simulink model "bh_smd_MAIN_HELLO"  (R2018a)
settings: Solver=ode45  StartTime=0.0  StopTime=10.0  RelTol=1e-7
settings Model: Creator=bhorton  LastModifiedBy=bhorton
settings CodeAppCC: StateflowObjectComments=on

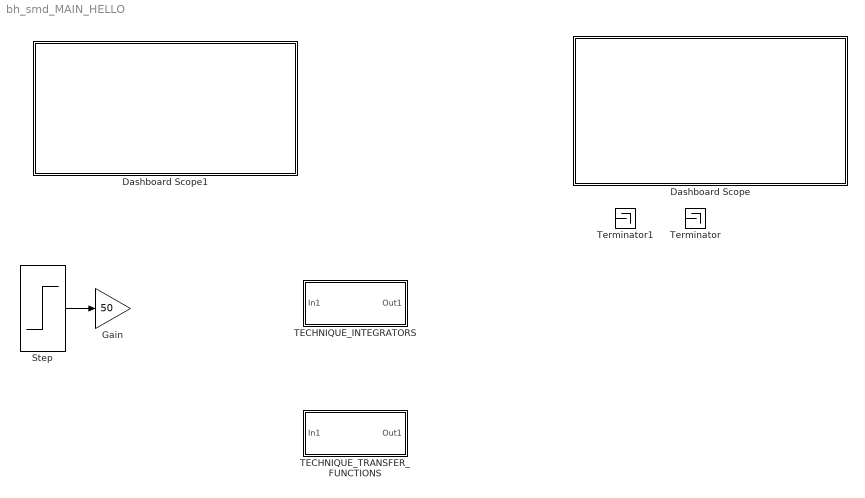
== system bh_smd_MAIN_HELLO ==
  Dashboard Scope : Subsystem  DialogController=hmiCreateDDGDialog  IsWebBlock=on  mask(MWDashboardBlock){webBlockId=47d7a76a-e090-4f37-bb13-c45fee118520, webBlockType=sdiscope, ShowInitialText=on, HMISrcModelName=bh_smd_MAIN_HELLO}
      mask prompts: webBlockId "WebBlock Id"; webBlockType "WebBlock Type"; HMISrcModelName "Source Model"
      mask help: SimulinkHMI:dialogs:HMIScopeDialogDesc
      mask Help: helpview([docroot '/mapfiles/simulink.map'], 'hmi_scope')
      mask Display:
      | if strcmp(get_param(bdroot(gcb),'BlockDiagramType'), 'library')
      |     image([(matlabroot) '/toolbox/simulink/hmi/icons/DashboardScope.png']);
      | end
  Dashboard Scope1 : Subsystem  DialogController=hmiCreateDDGDialog  IsWebBlock=on  mask(MWDashboardBlock){webBlockId=8ddedbd7-6b40-4d71-b8ad-862d34055e22, webBlockType=sdiscope, ShowInitialText=on, HMISrcModelName=bh_smd_MAIN_HELLO}
      mask prompts: webBlockId "WebBlock Id"; webBlockType "WebBlock Type"; HMISrcModelName "Source Model"
      mask help: SimulinkHMI:dialogs:HMIScopeDialogDesc
      mask Help: helpview([docroot '/mapfiles/simulink.map'], 'hmi_scope')
      mask Display:
      | if strcmp(get_param(bdroot(gcb),'BlockDiagramType'), 'library')
      |     image([(matlabroot) '/toolbox/simulink/hmi/icons/DashboardScope.png']);
      | end
  Gain : Gain  Gain=50
  Step : Step  Time=5  SampleTime=0
  TECHNIQUE_INTEGRATORS : Subsystem
  TECHNIQUE_TRANSFER_FUNCTIONS : Subsystem
  Terminator : Terminator
  Terminator1 : Terminator
  wires:
  Step/1 -> Gain/1

== system bh_smd_MAIN_HELLO/Dashboard Scope ==

== system bh_smd_MAIN_HELLO/Dashboard Scope1 ==

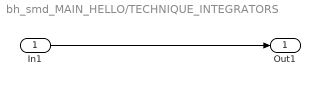
== system bh_smd_MAIN_HELLO/TECHNIQUE_INTEGRATORS ==
  In1 : Inport
  Out1 : Outport
  wires:
  In1/1 -> Out1/1

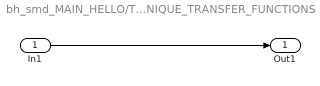
== system bh_smd_MAIN_HELLO/TECHNIQUE_TRANSFER_FUNCTIONS ==
  In1 : Inport
  Out1 : Outport
  wires:
  In1/1 -> Out1/1
